simulink model "mpmsm_model"  (R2015b)
settings: Solver=ode45  StartTime=0.0  StopTime=0.04  RelTol=1e-3
values from neighbouring files (symbols this model uses):
  EA = expm(A*T)    [init.m]
  Fm = 1.25/p    (= 0.0833333333333)    [init.m]
  J = 0.0001    [init.m]
  Kv = 0.1/p    (= 0.00666666666667)    [init.m]
  Ls = 0.001    [init.m]
  p = 15    [init.m]
  Rs = 0.5    [init.m]
  T = 0.001    [init.m]
undefined symbols (not defined in the file or in its folder): pmsm_dmodel, pmsm_model
settings Model: Creator=Andrey  LastModifiedBy=Andrey

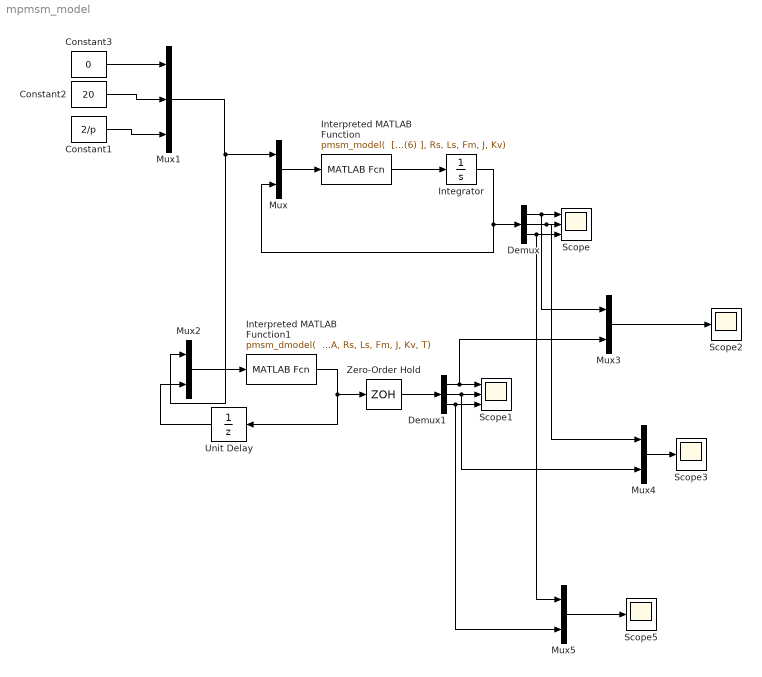
== system mpmsm_model ==
  Constant1 : Constant  Value=2/p
  Constant2 : Constant  Value=20
  Constant3 : Constant  Value=0
  Demux : Demux  Outputs=3
  Demux1 : Demux  Outputs=3
  Integrator : Integrator  InitialCondition=[0,0,0]
  Interpreted MATLAB Function : MATLABFcn  MATLABFcn="pmsm_model(  [u(1) u(2) u(3)], [u(4) u(5) u(6) ], Rs, Ls, Fm, J, Kv)"  OutputDimensions=3
  Interpreted MATLAB Function1 : MATLABFcn  MATLABFcn="pmsm_dmodel(  [u(1) u(2) u(3)], [u(4) u(5) u(6) ], EA, Rs, Ls, Fm, J, Kv, T)"  OutputDimensions=3
  Mux{,2..5} (5 alike) : Mux  Inputs=2
  Mux1 : Mux  Inputs=3
  Scope : Scope  NumInputPorts=3
  Scope1 : Scope  NumInputPorts=3
  Scope2 : Scope
  Scope3 : Scope
  Scope5 : Scope
  Unit Delay : UnitDelay  InitialCondition=[0 0 0]  SampleTime=T
  Zero-Order Hold : ZeroOrderHold  SampleTime=T
  wires:
  Mux/1 -> Interpreted MATLAB Function/1
  Integrator/1 -> Demux/1, Mux/2
  Mux1/1 -> Mux2/1, Mux/1
  Constant1/1 -> Mux1/3
  Interpreted MATLAB Function/1 -> Integrator/1
  Constant2/1 -> Mux1/2
  Demux/1 -> Mux3/1, Scope/1
  Demux/2 -> Mux4/1, Scope/2
  Demux/3 -> Mux5/1, Scope/3
  Constant3/1 -> Mux1/1
  Mux2/1 -> Interpreted MATLAB Function1/1
  Interpreted MATLAB Function1/1 -> Unit Delay/1, Zero-Order Hold/1
  Demux1/1 -> Mux3/2, Scope1/1
  Demux1/2 -> Mux4/2, Scope1/2
  Demux1/3 -> Mux5/2, Scope1/3
  Unit Delay/1 -> Mux2/2
  Mux3/1 -> Scope2/1
  Mux4/1 -> Scope3/1
  Mux5/1 -> Scope5/1
  Zero-Order Hold/1 -> Demux1/1
